simulink model "exampleModel_bus_axi"  (R2017b)
settings: Solver=VariableStepAuto  StartTime=0.0  StopTime=3e-5  RelTol=1e-3
PreLoadFcn:
  | setup
values from neighbouring files (symbols this model uses):
  axiClk = 156.25e6    (= 156250000)    [setup.m]    (also in setup_exampleModel_bus_axi_simulink.m; setup_exampleModel_bus_axi_simulink_lcls2.m; setup_lcls2_pcav.m; sysgen_signal.m)
  cav1p1_addr = 204    [setup_exampleModel_bus_axi_simulink.m]    (also in setup_exampleModel_bus_axi_simulink_lcls2.m; setup_lcls2_pcav.m; sysgen_signal.m)
  cav1p2_addr = cav1p1_addr * 2    (= 408)    [setup_exampleModel_bus_axi_simulink.m]    (also in setup_exampleModel_bus_axi_simulink_lcls2.m; setup_lcls2_pcav.m; sysgen_signal.m)
  cav2p1_addr = cav1p1_addr * 3    (= 612)    [setup_exampleModel_bus_axi_simulink.m]    (also in setup_exampleModel_bus_axi_simulink_lcls2.m; setup_lcls2_pcav.m; sysgen_signal.m)
  cav2p2_addr = cav1p1_addr * 4    (= 816)    [setup_exampleModel_bus_axi_simulink.m]    (also in setup_exampleModel_bus_axi_simulink_lcls2.m; setup_lcls2_pcav.m; sysgen_signal.m)
  Fadc = Fs/interleavedChannels    (= 29750000)    [setup.m]    (also in setup_exampleModel_bus_axi_simulink.m = 357000000; setup_exampleModel_bus_axi_simulink_lcls2.m = 351000000; setup_lcls2_pcav.m = 357000000; sysgen_signal.m = 357000000)
  Fproc = 204e6    (= 204000000)    [setup_exampleModel_bus_axi_simulink.m]    (also in setup_exampleModel_bus_axi_simulink_lcls2.m = 200571400; setup_lcls2_pcav.m; sysgen_signal.m)
  Fsig = Fproc/12    (= 17000000)    [setup_exampleModel_bus_axi_simulink.m]    (also in setup_exampleModel_bus_axi_simulink_lcls2.m = 16714283.3333; setup_lcls2_pcav.m)
  Tadc = 1/fadc    (= 2.80112044818e-09)    [cavity_signal.m]    (also in setup_exampleModel_bus_axi_simulink.m; setup_exampleModel_bus_axi_simulink_lcls2.m = 2.849002849e-09; setup_lcls2_pcav.m; setup_pcav_simulink.m)
undefined symbols (not defined in the file or in its folder): AXI4, Lite
libraries: xbsIndex_r4 x2037, llrf_lib x10, simulink x1
(part 6 of 12)

== system exampleModel_bus_axi/example/dsp/Cav1/Masking_n_delay ==
  note: delay for the comparison because Axilite register
      | takes a about 40 dsp clk cycles to load in
  phi_reset_trig : Inport
  start_pt : Inport  Port=2
  stop_pt : Inport  Port=3
  flo_start : Inport  Port=4
  flo_stop : Inport  Port=5
  Constant1 : xbsIndex_r4/Constant  const=0  gui_display_data_type=Fixed-point  arith_type=Unsigned  n_bits=16  bin_pt=0  preci_type=Single  exp_width=8  frac_width=24  explicit_period=off  period=1  equ=P=C  opselect=C  inp2=PCIN>>17  opr=+  inp1=P  carry=CIN  dbl_ovrd=off  block_type=constant
  Constant4 : xbsIndex_r4/Constant  const=0  gui_display_data_type=Fixed-point  arith_type=Unsigned  n_bits=1  bin_pt=0  preci_type=Single  exp_width=8  frac_width=24  explicit_period=off  period=1  equ=P=C  opselect=C  inp2=PCIN>>17  opr=+  inp1=P  carry=CIN  dbl_ovrd=off  block_type=constant
  Convert11 : xbsIndex_r4/Convert  gui_display_data_type=Fixed-point  arith_type=Unsigned  n_bits=1  bin_pt=0  float_type=Single  exp_bits=8  fraction_bits=24  quantization=Truncate  overflow=Wrap  en=off  latency=1  pipeline=off  dbl_ovrd=off  block_type=convert
  Convert2 : xbsIndex_r4/Convert  gui_display_data_type=Fixed-point  arith_type=Unsigned  n_bits=1  bin_pt=0  float_type=Single  exp_bits=8  fraction_bits=24  quantization=Truncate  overflow=Wrap  en=off  latency=1  pipeline=off  dbl_ovrd=off  block_type=convert
  Convert3 : xbsIndex_r4/Convert  gui_display_data_type=Boolean  arith_type=Boolean  n_bits=16  bin_pt=14  float_type=Single  exp_bits=8  fraction_bits=24  quantization=Truncate  overflow=Wrap  en=off  latency=1  pipeline=off  dbl_ovrd=off  block_type=convert
  Convert4 : xbsIndex_r4/Convert  gui_display_data_type=Fixed-point  arith_type=Unsigned  n_bits=8  bin_pt=0  float_type=Single  exp_bits=8  fraction_bits=24  quantization=Truncate  overflow=Saturate  en=off  latency=1  pipeline=off  dbl_ovrd=off  block_type=convert
  Convert7 : xbsIndex_r4/Convert  gui_display_data_type=Boolean  arith_type=Boolean  n_bits=1  bin_pt=0  float_type=Single  exp_bits=8  fraction_bits=24  quantization=Truncate  overflow=Wrap  en=off  latency=1  pipeline=off  dbl_ovrd=off  block_type=convert
  Convert8 : xbsIndex_r4/Convert  gui_display_data_type=Boolean  arith_type=Boolean  n_bits=1  bin_pt=0  float_type=Single  exp_bits=8  fraction_bits=24  quantization=Truncate  overflow=Wrap  en=off  latency=1  pipeline=off  dbl_ovrd=off  block_type=convert
  Counter : xbsIndex_r4/Counter  cnt_type=Count Limited  cnt_to=2^15  operation=Up  start_count=0  cnt_by_val=1  arith_type=Unsigned  n_bits=16  bin_pt=0  load_pin=off  rst=on  en=on  explicit_period=off  period=12/Fproc  use_behavioral_HDL=off  implementation=Fabric  dbl_ovrd=off  block_type=counter
  Delay{1..4} (4 alike) : xbsIndex_r4/Delay  rst=off  infoeditControl=Selection of Reset will increase slice count due to use of real FFs and instead of SRLs  en=off  latency=1  reg_retiming=off  dbl_ovrd=off  block_type=delay
  Delay6 : xbsIndex_r4/Delay  rst=off  infoeditControl=Selection of Reset will increase slice count due to use of real FFs and instead of SRLs  en=off  latency=2  reg_retiming=off  dbl_ovrd=off  block_type=delay
  Delay7 : xbsIndex_r4/Delay  rst=off  infoeditControl=Selection of Reset will increase slice count due to use of real FFs and instead of SRLs  en=off  latency=2  reg_retiming=off  dbl_ovrd=off  block_type=delay
  Down Sample{1..4} (4 alike) : xbsIndex_r4/Down Sample  sample_ratio=12  sample_phase="Last Value of Frame  (most efficient)"  en=off  rst=off  latency=1  dbl_ovrd=off  block_type=dsamp
  Logical1 : xbsIndex_r4/Logical  logical_function=AND  inputs=2  en=off  latency=1  precision=Full  arith_type=Unsigned  n_bits=16  bin_pt=0  align_bp=on  dbl_ovrd=off  block_type=logical
  Logical2 : xbsIndex_r4/Logical  logical_function=AND  inputs=2  en=off  latency=1  precision=Full  arith_type=Unsigned  n_bits=16  bin_pt=0  align_bp=on  dbl_ovrd=off  block_type=logical
  Register1 : xbsIndex_r4/Register  init=0  rst=off  en=on  dbl_ovrd=off  block_type=register
  Register10 : xbsIndex_r4/Register  init=0  rst=off  en=off  dbl_ovrd=off  block_type=register
  Register2 : xbsIndex_r4/Register  init=100  rst=off  en=off  dbl_ovrd=off  block_type=register
  Register3 : xbsIndex_r4/Register  init=100  rst=off  en=off  dbl_ovrd=off  block_type=register
  Register5 : xbsIndex_r4/Register  init=0  rst=off  en=off  dbl_ovrd=off  block_type=register
  Register6 : xbsIndex_r4/Register  init=100  rst=off  en=off  dbl_ovrd=off  block_type=register
  Relational1 : xbsIndex_r4/Relational  mode=a<b  op_type=Bool  en=on  latency=1  dbl_ovrd=off  block_type=relational
  Relational2 : xbsIndex_r4/Relational  mode=a>b  op_type=Bool  en=off  latency=1  dbl_ovrd=off  block_type=relational
  Relational3 : xbsIndex_r4/Relational  mode=a<b  op_type=Bool  en=on  latency=1  dbl_ovrd=off  block_type=relational
  Relational4 : xbsIndex_r4/Relational  mode=a>b  op_type=Bool  en=on  latency=1  dbl_ovrd=off  block_type=relational
  Relational6 : xbsIndex_r4/Relational  mode=a>b  op_type=Bool  en=on  latency=1  dbl_ovrd=off  block_type=relational
  Relational7 : xbsIndex_r4/Relational  mode=a>b  op_type=Bool  en=off  latency=1  dbl_ovrd=off  block_type=relational
  trig_reset : Outport
  counter : Outport  Port=2
  eval_window : Outport  Port=3
  flo_window : Outport  Port=4
  Stream_valid : Outport  Port=5
  wires:
  start_pt/1 -> Register5/1
  phi_reset_trig/1 -> Register10/1
  Register5/1 -> Down Sample1/1
  stop_pt/1 -> Register6/1
  Register6/1 -> Down Sample2/1
  Convert3/1 -> Register1/2, Register1/1, Counter/1, trig_reset/1
  Delay2/1 -> Relational4/2
  Delay3/1 -> Relational3/2
  Constant1/1 -> Relational2/2
  Relational3/1 -> Convert7/1
  Relational4/1 -> Convert8/1
  Logical1/1 -> Convert11/1
  Convert8/1 -> Logical1/1
  Convert7/1 -> Logical1/2
  Convert11/1 -> eval_window/1
  Relational2/1 -> [enb], Relational3/3, Relational4/3
  Counter/1 -> Convert4/1
  Down Sample1/1 -> Delay2/1
  Down Sample2/1 -> [stop], Delay3/1
  Delay1/1 -> Relational4/1
  Delay4/1 -> Relational3/1
  Delay7/1 -> Relational1/1
  flo_stop/1 -> Register3/1
  Logical2/1 -> Convert2/1
  Relational1/1 -> Logical2/2
  Convert2/1 -> flo_window/1
  Delay6/1 -> Relational6/1
  flo_start/1 -> Register2/1
  Relational6/1 -> Logical2/1
  Constant4/1 -> Relational7/2
  Relational7/1 -> Stream_valid/1
  Register10/1 -> Convert3/1
  Register1/1 -> Counter/2
  Convert4/1 -> [cntr], Relational7/1, counter/1
  [cntr] -> Relational2/1, Delay4/1, Delay1/1
  [cntr] -> Delay7/1, Delay6/1
  [enb] -> Relational6/3, Relational1/3
  Register2/1 -> Down Sample3/1
  Down Sample3/1 -> Relational6/2
  Down Sample4/1 -> Relational1/2
  Register3/1 -> Down Sample4/1

== system exampleModel_bus_axi/example/dsp/Cav1/PA_select ==
  PA_bus : Inport
  PA_chan_sel : Inport  Port=2
  Bus Creator3 : BusCreator  Inputs=3
  Bus Selector : BusSelector  OutputSignals=amp,phase,sync
  Bus Selector1 : BusSelector  OutputSignals=amp,phase,sync,channel
  Channel Select1 : llrf_lib/Sysgen/Single Rate/Channel Select  SystemSampleTime=-1
      settings: SourceProductName=LLRF Library
  Amp : Outport
  Phase : Outport  Port=2
  sync : Outport  Port=3
  wires:
  Bus Selector/3 -> sync/1  "<sync>"
  Bus Selector/2 -> Phase/1  "<phase>"
  Bus Selector/1 -> Amp/1  "<amp>"
  Bus Selector1/1 -> Channel Select1/1  "<amp>"
  Bus Selector1/2 -> Channel Select1/2  "<phase>"
  Bus Selector1/3 -> Channel Select1/3  "<sync>"
  Bus Selector1/4 -> Channel Select1/4  "<channel>"
  Channel Select1/1 -> Bus Creator3/1  "amp"
  Channel Select1/2 -> Bus Creator3/2  "phase"
  Channel Select1/3 -> Bus Creator3/3  "sync"
  Bus Creator3/1 -> Bus Selector/1
  PA_chan_sel/1 -> Channel Select1/5
  PA_bus/1 -> Bus Selector1/1

== system exampleModel_bus_axi/example/dsp/Cav1/PA_select1 ==
  PA_bus : Inport
  PA_chan_sel : Inport  Port=2
  Bus Creator3 : BusCreator  Inputs=3
  Bus Selector : BusSelector  OutputSignals=amp,phase,sync
  Bus Selector1 : BusSelector  OutputSignals=amp,phase,sync,channel
  Channel Select1 : llrf_lib/Sysgen/Single Rate/Channel Select  SystemSampleTime=-1
      settings: SourceProductName=LLRF Library
  Amp : Outport
  Phase : Outport  Port=2
  sync : Outport  Port=3
  wires:
  PA_bus/1 -> Bus Selector1/1
  PA_chan_sel/1 -> Channel Select1/5
  Bus Creator3/1 -> Bus Selector/1
  Channel Select1/3 -> Bus Creator3/3  "sync"
  Channel Select1/2 -> Bus Creator3/2  "phase"
  Channel Select1/1 -> Bus Creator3/1  "amp"
  Bus Selector1/4 -> Channel Select1/4  "<channel>"
  Bus Selector1/3 -> Channel Select1/3  "<sync>"
  Bus Selector1/2 -> Channel Select1/2  "<phase>"
  Bus Selector1/1 -> Channel Select1/1  "<amp>"
  Bus Selector/1 -> Amp/1  "<amp>"
  Bus Selector/2 -> Phase/1  "<phase>"
  Bus Selector/3 -> sync/1  "<sync>"

== system exampleModel_bus_axi/example/dsp/Cav1/Subsystem1 ==
  IQ_stream_in : Inport
  IQ_chan_sel : Inport  Port=2
  Bus Creator5 : BusCreator  Inputs=3
  Bus Selector : BusSelector  OutputSignals=ddcI,ddcQ,sync
  Bus Selector3 : BusSelector  OutputSignals=ddcI,ddcQ,ddcSync,ddcChannel
  Channel Select3 : llrf_lib/Sysgen/Single Rate/Channel Select  SystemSampleTime=-1
      settings: SourceProductName=LLRF Library
  ddcI : Outport
  ddcQ : Outport  Port=2
  sync : Outport  Port=3
  wires:
  IQ_stream_in/1 -> Bus Selector3/1
  IQ_chan_sel/1 -> Channel Select3/5
  Channel Select3/3 -> Bus Creator5/3  "sync"
  Bus Selector3/2 -> Channel Select3/2  "<ddcQ>"
  Channel Select3/1 -> Bus Creator5/1  "ddcI"
  Channel Select3/2 -> Bus Creator5/2  "ddcQ"
  Bus Selector3/1 -> Channel Select3/1  "<ddcI>"
  Bus Selector3/4 -> Channel Select3/4  "<ddcChannel>"
  Bus Selector3/3 -> Channel Select3/3  "<ddcSync>"
  Bus Creator5/1 -> Bus Selector/1
  Bus Selector/1 -> ddcI/1  "<ddcI>"
  Bus Selector/2 -> ddcQ/1  "<ddcQ>"
  Bus Selector/3 -> sync/1  "<sync>"

== system exampleModel_bus_axi/example/dsp/Cav1/Subsystem10 ==
  d : Inport
  reset : Inport  Port=2
  cntr : Inport  Port=3
  threshold : Inport  Port=4
  Register11 : xbsIndex_r4/Register  init=0  rst=on  en=on  dbl_ovrd=off  block_type=register
  Relational4 : xbsIndex_r4/Relational  mode=a>b  op_type=Bool  en=off  latency=1  dbl_ovrd=off  block_type=relational
  posedge_pulse : Subsystem
  q : Outport
  wires:
  threshold/1 -> Relational4/2
  reset/1 -> Register11/2
  Relational4/1 -> posedge_pulse/1(In1)
  posedge_pulse/1(Out1) -> Register11/3
  Register11/1 -> q/1
  cntr/1 -> Relational4/1
  d/1 -> Register11/1

== system exampleModel_bus_axi/example/dsp/Cav1/Subsystem11 ==
  d : Inport
  reset : Inport  Port=2
  cntr : Inport  Port=3
  threshold : Inport  Port=4
  Register11 : xbsIndex_r4/Register  init=0  rst=on  en=on  dbl_ovrd=off  block_type=register
  Relational4 : xbsIndex_r4/Relational  mode=a>b  op_type=Bool  en=off  latency=1  dbl_ovrd=off  block_type=relational
  posedge_pulse : Subsystem
  q : Outport
  wires:
  d/1 -> Register11/1
  cntr/1 -> Relational4/1
  Register11/1 -> q/1
  posedge_pulse/1(Out1) -> Register11/3
  Relational4/1 -> posedge_pulse/1(In1)
  reset/1 -> Register11/2
  threshold/1 -> Relational4/2

== system exampleModel_bus_axi/example/dsp/Cav1/Subsystem12 ==
  d : Inport
  reset : Inport  Port=2
  cntr : Inport  Port=3
  threshold : Inport  Port=4
  Register11 : xbsIndex_r4/Register  init=0  rst=on  en=on  dbl_ovrd=off  block_type=register
  Relational4 : xbsIndex_r4/Relational  mode=a>b  op_type=Bool  en=off  latency=1  dbl_ovrd=off  block_type=relational
  posedge_pulse : Subsystem
  q : Outport
  wires:
  threshold/1 -> Relational4/2
  reset/1 -> Register11/2
  Relational4/1 -> posedge_pulse/1(In1)
  posedge_pulse/1(Out1) -> Register11/3
  Register11/1 -> q/1
  cntr/1 -> Relational4/1
  d/1 -> Register11/1

== system exampleModel_bus_axi/example/dsp/Cav1/Subsystem13 ==
  d : Inport
  reset : Inport  Port=2
  cntr : Inport  Port=3
  threshold : Inport  Port=4
  Register11 : xbsIndex_r4/Register  init=0  rst=on  en=on  dbl_ovrd=off  block_type=register
  Relational4 : xbsIndex_r4/Relational  mode=a>b  op_type=Bool  en=off  latency=1  dbl_ovrd=off  block_type=relational
  posedge_pulse : Subsystem
  q : Outport
  wires:
  d/1 -> Register11/1
  cntr/1 -> Relational4/1
  Register11/1 -> q/1
  posedge_pulse/1(Out1) -> Register11/3
  Relational4/1 -> posedge_pulse/1(In1)
  reset/1 -> Register11/2
  threshold/1 -> Relational4/2

== system exampleModel_bus_axi/example/dsp/Cav1/Subsystem14 ==
  d : Inport
  reset : Inport  Port=2
  cntr : Inport  Port=3
  threshold : Inport  Port=4
  Register11 : xbsIndex_r4/Register  init=0  rst=on  en=on  dbl_ovrd=off  block_type=register
  Relational4 : xbsIndex_r4/Relational  mode=a>b  op_type=Bool  en=off  latency=1  dbl_ovrd=off  block_type=relational
  posedge_pulse : Subsystem
  q : Outport
  wires:
  threshold/1 -> Relational4/2
  reset/1 -> Register11/2
  Relational4/1 -> posedge_pulse/1(In1)
  posedge_pulse/1(Out1) -> Register11/3
  Register11/1 -> q/1
  cntr/1 -> Relational4/1
  d/1 -> Register11/1

== system exampleModel_bus_axi/example/dsp/Cav1/Subsystem2 ==
  d : Inport
  reset : Inport  Port=2
  cntr : Inport  Port=3
  threshold : Inport  Port=4
  Register11 : xbsIndex_r4/Register  init=0  rst=on  en=on  dbl_ovrd=off  block_type=register
  Relational4 : xbsIndex_r4/Relational  mode=a>b  op_type=Bool  en=off  latency=1  dbl_ovrd=off  block_type=relational
  posedge_pulse : Subsystem
  q : Outport
  wires:
  d/1 -> Register11/1
  cntr/1 -> Relational4/1
  Register11/1 -> q/1
  posedge_pulse/1(Out1) -> Register11/3
  Relational4/1 -> posedge_pulse/1(In1)
  reset/1 -> Register11/2
  threshold/1 -> Relational4/2

== system exampleModel_bus_axi/example/dsp/Cav1/Subsystem3 ==
  IQ_stream_in : Inport
  IQ_chan_sel : Inport  Port=2
  Bus Creator5 : BusCreator  Inputs=3
  Bus Selector : BusSelector  OutputSignals=ddcI,ddcQ,sync
  Bus Selector3 : BusSelector  OutputSignals=ddcI,ddcQ,ddcSync,ddcChannel
  Channel Select3 : llrf_lib/Sysgen/Single Rate/Channel Select  SystemSampleTime=-1
      settings: SourceProductName=LLRF Library
  ddcI : Outport
  ddcQ : Outport  Port=2
  sync : Outport  Port=3
  wires:
  Bus Selector/3 -> sync/1  "<sync>"
  Bus Selector/2 -> ddcQ/1  "<ddcQ>"
  Bus Selector/1 -> ddcI/1  "<ddcI>"
  Bus Creator5/1 -> Bus Selector/1
  Bus Selector3/3 -> Channel Select3/3  "<ddcSync>"
  Bus Selector3/4 -> Channel Select3/4  "<ddcChannel>"
  Bus Selector3/1 -> Channel Select3/1  "<ddcI>"
  Channel Select3/2 -> Bus Creator5/2  "ddcQ"
  Channel Select3/1 -> Bus Creator5/1  "ddcI"
  Bus Selector3/2 -> Channel Select3/2  "<ddcQ>"
  Channel Select3/3 -> Bus Creator5/3  "sync"
  IQ_chan_sel/1 -> Channel Select3/5
  IQ_stream_in/1 -> Bus Selector3/1

== system exampleModel_bus_axi/example/dsp/Cav1/Subsystem4 ==
  d : Inport
  reset : Inport  Port=2
  cntr : Inport  Port=3
  threshold : Inport  Port=4
  Gateway Out{1,7..9} (4 alike) : xbsIndex_r4/Gateway Out  inherit_from_input=off  hdl_port=on  rows=1  columns=1  UseAsDAC=off  DACChannel='1'  interface=None  automatic_assignment=on  address_offset=hex2dec('00')  intf_name=''  intf_description=''  timing_constraint=None  locs_specified=off  LOCs={}  io_standard={}  block_type=gatewayout
  Register11 : xbsIndex_r4/Register  init=0  rst=on  en=on  dbl_ovrd=off  block_type=register
  Relational4 : xbsIndex_r4/Relational  mode=a>b  op_type=Bool  en=off  latency=1  dbl_ovrd=off  block_type=relational
  Scope3 : Scope  NumInputPorts=4
  posedge_pulse : Subsystem
  q : Outport
  wires:
  d/1 -> Gateway Out7/1, Register11/1
  cntr/1 -> Relational4/1
  Register11/1 -> Gateway Out8/1, q/1
  posedge_pulse/1(Out1) -> Register11/3, Gateway Out1/1
  Relational4/1 -> posedge_pulse/1(In1)
  reset/1 -> Gateway Out9/1, Register11/2
  threshold/1 -> Relational4/2
  Gateway Out1/1 -> Scope3/4
  Gateway Out7/1 -> Scope3/1
  Gateway Out8/1 -> Scope3/2
  Gateway Out9/1 -> Scope3/3

== system exampleModel_bus_axi/example/dsp/Cav1/Subsystem5 ==
  d : Inport
  reset : Inport  Port=2
  cntr : Inport  Port=3
  threshold : Inport  Port=4
  Register11 : xbsIndex_r4/Register  init=0  rst=on  en=on  dbl_ovrd=off  block_type=register
  Relational4 : xbsIndex_r4/Relational  mode=a>b  op_type=Bool  en=off  latency=1  dbl_ovrd=off  block_type=relational
  posedge_pulse : Subsystem
  q : Outport
  wires:
  threshold/1 -> Relational4/2
  reset/1 -> Register11/2
  Relational4/1 -> posedge_pulse/1(In1)
  posedge_pulse/1(Out1) -> Register11/3
  Register11/1 -> q/1
  cntr/1 -> Relational4/1
  d/1 -> Register11/1

== system exampleModel_bus_axi/example/dsp/Cav1/Subsystem6 ==
  d : Inport
  reset : Inport  Port=2
  cntr : Inport  Port=3
  threshold : Inport  Port=4
  Register11 : xbsIndex_r4/Register  init=0  rst=on  en=on  dbl_ovrd=off  block_type=register
  Relational4 : xbsIndex_r4/Relational  mode=a>b  op_type=Bool  en=off  latency=1  dbl_ovrd=off  block_type=relational
  posedge_pulse : Subsystem
  q : Outport
  wires:
  threshold/1 -> Relational4/2
  reset/1 -> Register11/2
  Relational4/1 -> posedge_pulse/1(In1)
  posedge_pulse/1(Out1) -> Register11/3
  Register11/1 -> q/1
  cntr/1 -> Relational4/1
  d/1 -> Register11/1

== system exampleModel_bus_axi/example/dsp/Cav1/Subsystem7 ==
  d : Inport
  reset : Inport  Port=2
  cntr : Inport  Port=3
  threshold : Inport  Port=4
  Register11 : xbsIndex_r4/Register  init=0  rst=on  en=on  dbl_ovrd=off  block_type=register
  Relational4 : xbsIndex_r4/Relational  mode=a>b  op_type=Bool  en=off  latency=1  dbl_ovrd=off  block_type=relational
  posedge_pulse : Subsystem
  q : Outport
  wires:
  d/1 -> Register11/1
  cntr/1 -> Relational4/1
  Register11/1 -> q/1
  posedge_pulse/1(Out1) -> Register11/3
  Relational4/1 -> posedge_pulse/1(In1)
  reset/1 -> Register11/2
  threshold/1 -> Relational4/2

== system exampleModel_bus_axi/example/dsp/Cav1/Subsystem8 ==
  d : Inport
  reset : Inport  Port=2
  cntr : Inport  Port=3
  threshold : Inport  Port=4
  Register11 : xbsIndex_r4/Register  init=0  rst=on  en=on  dbl_ovrd=off  block_type=register
  Relational4 : xbsIndex_r4/Relational  mode=a>b  op_type=Bool  en=off  latency=1  dbl_ovrd=off  block_type=relational
  posedge_pulse : Subsystem
  q : Outport
  wires:
  threshold/1 -> Relational4/2
  reset/1 -> Register11/2
  Relational4/1 -> posedge_pulse/1(In1)
  posedge_pulse/1(Out1) -> Register11/3
  Register11/1 -> q/1
  cntr/1 -> Relational4/1
  d/1 -> Register11/1

== system exampleModel_bus_axi/example/dsp/Cav1/Subsystem9 ==
  d : Inport
  reset : Inport  Port=2
  cntr : Inport  Port=3
  threshold : Inport  Port=4
  Register11 : xbsIndex_r4/Register  init=0  rst=on  en=on  dbl_ovrd=off  block_type=register
  Relational4 : xbsIndex_r4/Relational  mode=a>b  op_type=Bool  en=off  latency=1  dbl_ovrd=off  block_type=relational
  posedge_pulse : Subsystem
  q : Outport
  wires:
  d/1 -> Register11/1
  cntr/1 -> Relational4/1
  Register11/1 -> q/1
  posedge_pulse/1(Out1) -> Register11/3
  Relational4/1 -> posedge_pulse/1(In1)
  reset/1 -> Register11/2
  threshold/1 -> Relational4/2

== system exampleModel_bus_axi/example/dsp/Cav1/c1p1_Masking_window ==
  note: delay for the comparison because Axilite register
      | takes a about 40 dsp clk cycles to load in
  counter : Inport
  start_pt : Inport  Port=2
  stop_pt : Inport  Port=3
  Constant1 : xbsIndex_r4/Constant  const=0  gui_display_data_type=Fixed-point  arith_type=Unsigned  n_bits=16  bin_pt=0  preci_type=Single  exp_width=8  frac_width=24  explicit_period=off  period=1  equ=P=C  opselect=C  inp2=PCIN>>17  opr=+  inp1=P  carry=CIN  dbl_ovrd=off  block_type=constant
  Convert11 : xbsIndex_r4/Convert  gui_display_data_type=Fixed-point  arith_type=Unsigned  n_bits=1  bin_pt=0  float_type=Single  exp_bits=8  fraction_bits=24  quantization=Truncate  overflow=Wrap  en=off  latency=1  pipeline=off  dbl_ovrd=off  block_type=convert
  Delay{1..4} (4 alike) : xbsIndex_r4/Delay  rst=off  infoeditControl=Selection of Reset will increase slice count due to use of real FFs and instead of SRLs  en=off  latency=1  reg_retiming=off  dbl_ovrd=off  block_type=delay
  Down Sample1 : xbsIndex_r4/Down Sample  sample_ratio=12  sample_phase="Last Value of Frame  (most efficient)"  en=off  rst=off  latency=1  dbl_ovrd=off  block_type=dsamp
  Down Sample2 : xbsIndex_r4/Down Sample  sample_ratio=12  sample_phase="Last Value of Frame  (most efficient)"  en=off  rst=off  latency=1  dbl_ovrd=off  block_type=dsamp
  Logical1 : xbsIndex_r4/Logical  logical_function=AND  inputs=2  en=off  latency=1  precision=Full  arith_type=Unsigned  n_bits=16  bin_pt=0  align_bp=on  dbl_ovrd=off  block_type=logical
  Register5 : xbsIndex_r4/Register  init=0  rst=off  en=off  dbl_ovrd=off  block_type=register
  Register6 : xbsIndex_r4/Register  init=100  rst=off  en=off  dbl_ovrd=off  block_type=register
  Relational2 : xbsIndex_r4/Relational  mode=a>b  op_type=Bool  en=off  latency=1  dbl_ovrd=off  block_type=relational
  Relational3 : xbsIndex_r4/Relational  mode=a<b  op_type=Bool  en=on  latency=1  dbl_ovrd=off  block_type=relational
  Relational4 : xbsIndex_r4/Relational  mode=a>b  op_type=Bool  en=on  latency=1  dbl_ovrd=off  block_type=relational
  eval_window : Outport
  wires:
  start_pt/1 -> Register5/1
  Register5/1 -> Down Sample1/1
  stop_pt/1 -> Register6/1
  Register6/1 -> Down Sample2/1
  Delay2/1 -> Relational4/2
  Delay3/1 -> [stop], Relational3/2
  Constant1/1 -> Relational2/2
  Logical1/1 -> Convert11/1
  Relational3/1 -> Logical1/2
  Convert11/1 -> eval_window/1
  Relational2/1 -> [enb], Relational3/3, Relational4/3
  counter/1 -> [cntr]
  Down Sample1/1 -> Delay2/1
  Down Sample2/1 -> Delay3/1
  Delay1/1 -> Relational4/1
  Delay4/1 -> Relational3/1
  Relational4/1 -> Logical1/1
  [cntr] -> Relational2/1, Delay1/1, Delay4/1

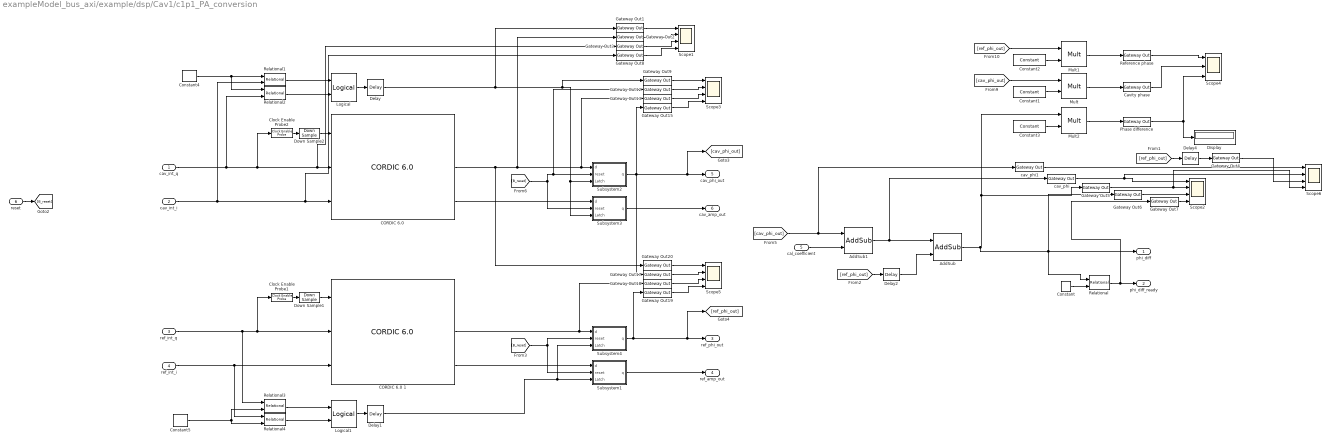
== system exampleModel_bus_axi/example/dsp/Cav1/c1p1_PA_conversion ==
  cav_int_q : Inport
  cav_int_i : Inport  Port=2
  ref_int_q : Inport  Port=3
  ref_int_i : Inport  Port=4
  cal_coefficient : Inport  Port=5
  reset : Inport  Port=6
  AddSub : xbsIndex_r4/AddSub  mode=Subtraction  use_carryin=off  use_carryout=off  en=off  latency=1  precision=User Defined  arith_type="Signed  (2's comp)"  n_bits=18  bin_pt=15  quantization=Truncate  overflow=Wrap  use_behavioral_HDL=off  hw_selection=Fabric  pipelined=off  dbl_ovrd=off  block_type=addsub
  AddSub1 : xbsIndex_r4/AddSub  mode=Addition  use_carryin=off  use_carryout=off  en=off  latency=1  precision=User Defined  arith_type="Signed  (2's comp)"  n_bits=18  bin_pt=15  quantization=Truncate  overflow=Wrap  use_behavioral_HDL=off  hw_selection=Fabric  pipelined=off  dbl_ovrd=off  block_type=addsub
  "CORDIC 6.0 " : xbsIndex_r4/CORDIC 6.0   functional_selection=Translate  architectural_configuration=Parallel  pipelining_mode=Maximum  data_format=SignedFraction  phase_format=Scaled_Radians  input_width=18  output_width=18  round_mode=Truncate  iterations=0  precision=0  compensation_scaling=No_Scale_Compensation  coarse_rotation=on  aclken=off  aresetn=off  out_tready=off  cartesian_has_tuser=off  cartesian_has_tlast=off  cartesian_tuser_width=1  phase_has_tuser=off  phase_has_tlast=off  phase_tuser_width=1  out_tlast_behv=Null  flow_control=NonBlocking  optimize_goal=Resources  trim_axipin_name=on  simulation_type=hybrid_sim  simulation_model=sysgen:cordic_v6_0  data_path_portlist={'s_axis_cartesian_tdata_imag', 's_axis_cartesian_tdata_real', 's_axis_phase_tdata_phase', 'm_axis_dout_tdata_imag', 'm_axis_dout_tdata_real', 'm_axis_dout_tdata_phase','m_axis_dout_tdata'}  ip_name=CORDIC  ip_version=6.0  dsptool_ready=true  ipcore_usecache=true  ipcore_useipmodelcache=true  wrapper_available=true  port_translation_map={ 'aclken' => 'en', 'aresetn' => 'rst' }  block_type=cordic_v6_0
      settings: infoedit=CORDIC 6.0
  CORDIC 6.0 1 : xbsIndex_r4/CORDIC 6.0   functional_selection=Translate  architectural_configuration=Parallel  pipelining_mode=Maximum  data_format=SignedFraction  phase_format=Scaled_Radians  input_width=18  output_width=18  round_mode=Truncate  iterations=0  precision=0  compensation_scaling=No_Scale_Compensation  coarse_rotation=on  aclken=off  aresetn=off  out_tready=off  cartesian_has_tuser=off  cartesian_has_tlast=off  cartesian_tuser_width=1  phase_has_tuser=off  phase_has_tlast=off  phase_tuser_width=1  out_tlast_behv=Null  flow_control=NonBlocking  optimize_goal=Resources  trim_axipin_name=on  simulation_type=hybrid_sim  simulation_model=sysgen:cordic_v6_0  data_path_portlist={'s_axis_cartesian_tdata_imag', 's_axis_cartesian_tdata_real', 's_axis_phase_tdata_phase', 'm_axis_dout_tdata_imag', 'm_axis_dout_tdata_real', 'm_axis_dout_tdata_phase','m_axis_dout_tdata'}  ip_name=CORDIC  ip_version=6.0  dsptool_ready=true  ipcore_usecache=true  ipcore_useipmodelcache=true  wrapper_available=true  port_translation_map={ 'aclken' => 'en', 'aresetn' => 'rst' }  block_type=cordic_v6_0
      settings: infoedit=CORDIC 6.0
  Cavity phase : xbsIndex_r4/Gateway Out  inherit_from_input=off  hdl_port=off  rows=1  columns=1  UseAsDAC=off  DACChannel='1'  interface=None  automatic_assignment=on  address_offset=hex2dec('00')  intf_name=''  intf_description=''  timing_constraint=None  locs_specified=off  LOCs={}  io_standard={}  block_type=gatewayout
  Clock Enable Probe1 : xbsIndex_r4/Clock Enable Probe  inherit_constraints=on  block_type=ceprobe
      settings: infoedit="Clock enable extractor.  Produces a Boolean output that mirrors the hardware clock enable associated with the input sample rate.<br><br>Hardware notes: in hardware this block costs nothing."
  Clock Enable Probe2 : xbsIndex_r4/Clock Enable Probe  inherit_constraints=on  block_type=ceprobe
      settings: infoedit="Clock enable extractor.  Produces a Boolean output that mirrors the hardware clock enable associated with the input sample rate.<br><br>Hardware notes: in hardware this block costs nothing."
  Constant : xbsIndex_r4/Constant  const=0  gui_display_data_type=Fixed-point  arith_type=Signed (2's comp)  n_bits=1  bin_pt=0  preci_type=Single  exp_width=8  frac_width=24  explicit_period=off  period=1  equ=P=C  opselect=C  inp2=PCIN>>17  opr=+  inp1=P  carry=CIN  dbl_ovrd=off  block_type=constant
  Constant1 : xbsIndex_r4/Constant  const=pi  gui_display_data_type=Fixed-point  arith_type=Unsigned  n_bits=16  bin_pt=14  preci_type=Single  exp_width=8  frac_width=24  explicit_period=off  period=1  equ=P=C  opselect=C  inp2=PCIN>>17  opr=+  inp1=P  carry=CIN  dbl_ovrd=off  block_type=constant
  Constant2 : xbsIndex_r4/Constant  const=pi  gui_display_data_type=Fixed-point  arith_type=Unsigned  n_bits=16  bin_pt=14  preci_type=Single  exp_width=8  frac_width=24  explicit_period=off  period=1  equ=P=C  opselect=C  inp2=PCIN>>17  opr=+  inp1=P  carry=CIN  dbl_ovrd=off  block_type=constant
  Constant3 : xbsIndex_r4/Constant  const=pi  gui_display_data_type=Fixed-point  arith_type=Unsigned  n_bits=16  bin_pt=14  preci_type=Single  exp_width=8  frac_width=24  explicit_period=off  period=1  equ=P=C  opselect=C  inp2=PCIN>>17  opr=+  inp1=P  carry=CIN  dbl_ovrd=off  block_type=constant
  Constant4 : xbsIndex_r4/Constant  const=0  gui_display_data_type=Fixed-point  arith_type=Signed (2's comp)  n_bits=16  bin_pt=14  preci_type=Single  exp_width=8  frac_width=24  explicit_period=off  period=1  equ=P=C  opselect=C  inp2=PCIN>>17  opr=+  inp1=P  carry=CIN  dbl_ovrd=off  block_type=constant
  Constant5 : xbsIndex_r4/Constant  const=0  gui_display_data_type=Fixed-point  arith_type=Signed (2's comp)  n_bits=16  bin_pt=14  preci_type=Single  exp_width=8  frac_width=24  explicit_period=off  period=1  equ=P=C  opselect=C  inp2=PCIN>>17  opr=+  inp1=P  carry=CIN  dbl_ovrd=off  block_type=constant
  Delay : xbsIndex_r4/Delay  rst=off  infoeditControl=Selection of Reset will increase slice count due to use of real FFs and instead of SRLs  en=off  latency=21  reg_retiming=off  dbl_ovrd=off  block_type=delay
  Delay1 : xbsIndex_r4/Delay  rst=off  infoeditControl=Selection of Reset will increase slice count due to use of real FFs and instead of SRLs  en=off  latency=21  reg_retiming=off  dbl_ovrd=off  block_type=delay
  Delay2 : xbsIndex_r4/Delay  rst=off  infoeditControl=Selection of Reset will increase slice count due to use of real FFs and instead of SRLs  en=off  latency=1  reg_retiming=off  dbl_ovrd=off  block_type=delay
  Delay4 : xbsIndex_r4/Delay  rst=off  infoeditControl=Selection of Reset will increase slice count due to use of real FFs and instead of SRLs  en=off  latency=1  reg_retiming=off  dbl_ovrd=off  block_type=delay
  Display : Display
  Down Sample1 : xbsIndex_r4/Down Sample  sample_ratio=12  sample_phase="Last Value of Frame  (most efficient)"  en=off  rst=off  latency=1  dbl_ovrd=off  block_type=dsamp
  Down Sample2 : xbsIndex_r4/Down Sample  sample_ratio=12  sample_phase="Last Value of Frame  (most efficient)"  en=off  rst=off  latency=1  dbl_ovrd=off  block_type=dsamp
  Gateway Out{1..9,12..13,15,17..20} (16 alike) : xbsIndex_r4/Gateway Out  inherit_from_input=off  hdl_port=off  rows=1  columns=1  UseAsDAC=off  DACChannel='1'  interface=None  automatic_assignment=on  address_offset=hex2dec('00')  intf_name=''  intf_description=''  timing_constraint=None  locs_specified=off  LOCs={}  io_standard={}  block_type=gatewayout
  Logical : xbsIndex_r4/Logical  logical_function=AND  inputs=2  en=off  latency=1  precision=Full  arith_type=Unsigned  n_bits=16  bin_pt=0  align_bp=on  dbl_ovrd=off  block_type=logical
  Logical1 : xbsIndex_r4/Logical  logical_function=AND  inputs=2  en=off  latency=1  precision=Full  arith_type=Unsigned  n_bits=16  bin_pt=0  align_bp=on  dbl_ovrd=off  block_type=logical
  Mult : xbsIndex_r4/Mult  precision=Full  arith_type="Signed  (2's comp)"  n_bits=16  bin_pt=14  quantization=Truncate  overflow=Wrap  en=off  latency=3  use_behavioral_HDL=off  opt=Speed  use_embedded=on  optimum_pipeline=off  pipeline=on  dbl_ovrd=off  use_rpm=on  placement_style=Triangular  block_type=mult
  Mult1 : xbsIndex_r4/Mult  precision=Full  arith_type="Signed  (2's comp)"  n_bits=16  bin_pt=14  quantization=Truncate  overflow=Wrap  en=off  latency=3  use_behavioral_HDL=off  opt=Speed  use_embedded=on  optimum_pipeline=off  pipeline=on  dbl_ovrd=off  use_rpm=on  placement_style=Triangular  block_type=mult
  Mult2 : xbsIndex_r4/Mult  precision=Full  arith_type="Signed  (2's comp)"  n_bits=16  bin_pt=14  quantization=Truncate  overflow=Wrap  en=off  latency=3  use_behavioral_HDL=off  opt=Speed  use_embedded=on  optimum_pipeline=off  pipeline=on  dbl_ovrd=off  use_rpm=on  placement_style=Triangular  block_type=mult
  Phase difference : xbsIndex_r4/Gateway Out  inherit_from_input=off  hdl_port=off  rows=1  columns=1  UseAsDAC=off  DACChannel='1'  interface=None  automatic_assignment=on  address_offset=hex2dec('00')  intf_name=''  intf_description=''  timing_constraint=None  locs_specified=off  LOCs={}  io_standard={}  block_type=gatewayout
  Reference phase : xbsIndex_r4/Gateway Out  inherit_from_input=off  hdl_port=off  rows=1  columns=1  UseAsDAC=off  DACChannel='1'  interface=None  automatic_assignment=on  address_offset=hex2dec('00')  intf_name=''  intf_description=''  timing_constraint=None  locs_specified=off  LOCs={}  io_standard={}  block_type=gatewayout
  Relational{,1..4} (5 alike) : xbsIndex_r4/Relational  mode=a!=b  op_type=Bool  en=off  latency=1  dbl_ovrd=off  block_type=relational
  Scope{1..3,5..6} (5 alike) : Scope  NumInputPorts=4
  Scope4 : Scope  NumInputPorts=3
  Subsystem1 : Subsystem
  Subsystem2 : Subsystem
  Subsystem3 : Subsystem
  Subsystem4 : Subsystem
  cav_phi : xbsIndex_r4/Gateway Out  inherit_from_input=off  hdl_port=off  rows=1  columns=1  UseAsDAC=off  DACChannel='1'  interface=None  automatic_assignment=on  address_offset=hex2dec('00')  intf_name=''  intf_description=''  timing_constraint=None  locs_specified=off  LOCs={}  io_standard={}  block_type=gatewayout
  cav_phi1 : xbsIndex_r4/Gateway Out  inherit_from_input=off  hdl_port=off  rows=1  columns=1  UseAsDAC=off  DACChannel='1'  interface=None  automatic_assignment=on  address_offset=hex2dec('00')  intf_name=''  intf_description=''  timing_constraint=None  locs_specified=off  LOCs={}  io_standard={}  block_type=gatewayout
  phi_diff : Outport
  phi_diff_ready : Outport  Port=2
  ref_phi_out : Outport  Port=3
  ref_amp_out : Outport  Port=4
  cav_phi_out : Outport  Port=5
  cav_amp_out : Outport  Port=6
  wires:
  ref_int_i/1 -> CORDIC 6.0 1/3, Relational4/1
  ref_int_q/1 -> Relational3/1, CORDIC 6.0 1/2, Clock Enable Probe1/1
  [ref_phi_out] -> Delay4/1
  AddSub1/1 -> cav_phi/1, AddSub/1
  [cav_phi_out] -> cav_phi1/1, AddSub1/1
  cal_coefficient/1 -> AddSub1/2
  Subsystem4/1(q) -> Gateway Out19/1, [ref_phi_out], ref_phi_out/1
  Subsystem1/1(q) -> ref_amp_out/1
  Subsystem2/1(q) -> Gateway Out17/1, Gateway Out15/1, [cav_phi_out], cav_phi_out/1
  Subsystem3/1(q) -> cav_amp_out/1
  reset/1 -> [B_reset]
  [B_reset] -> Subsystem4/2(reset), Subsystem1/2(reset)
  [B_reset] -> Subsystem3/2(reset), Gateway Out12/1, Subsystem2/2(reset)
  AddSub/1 -> Gateway Out6/1, phi_diff/1, Relational/1, Mult2/1, Gateway Out5/1
  Delay2/1 -> AddSub/2
  Gateway Out5/1 -> Scope6/4, Scope2/2
  cav_phi/1 -> Scope6/2, Scope2/1
  Gateway Out6/1 -> Scope2/3
  Gateway Out7/1 -> Scope2/4
  Constant/1 -> Relational/2
  Relational/1 -> Gateway Out7/1, phi_diff_ready/1
  Constant1/1 -> Mult/2
  [cav_phi_out] -> Mult/1
  [ref_phi_out] -> Mult1/1
  Constant2/1 -> Mult1/2
  Mult1/1 -> Reference phase/1
  Mult/1 -> Cavity phase/1
  Mult2/1 -> Phase difference/1
  Constant3/1 -> Mult2/2
  Cavity phase/1 -> Scope4/2
  Reference phase/1 -> Scope4/1
  Phase difference/1 -> Display/1, Scope4/3
  Clock Enable Probe2/1 -> Down Sample2/1
  Down Sample2/1 -> "CORDIC 6.0 "/1
  cav_int_q/1 -> Relational2/2, Clock Enable Probe2/1, Gateway Out3/1, "CORDIC 6.0 "/2
  Logical/1 -> Delay/1
  Relational2/1 -> Logical/2
  Relational1/1 -> Logical/1
  cav_int_i/1 -> Relational1/2, Gateway Out8/1, "CORDIC 6.0 "/3
  Constant4/1 -> Relational2/1, Relational1/1
  Delay/1 -> Gateway Out1/1, Gateway Out9/1, Subsystem3/3(Latch), Subsystem2/3(Latch)
  Clock Enable Probe1/1 -> Down Sample1/1
  Down Sample1/1 -> CORDIC 6.0 1/1
  Delay1/1 -> Subsystem4/3(Latch), Subsystem1/3(Latch)
  Relational3/1 -> Logical1/1
  Relational4/1 -> Logical1/2
  Logical1/1 -> Delay1/1
  Constant5/1 -> Relational4/2, Relational3/2
  CORDIC 6.0 1/3 -> Subsystem1/1(d)
  CORDIC 6.0 1/2 -> Gateway Out18/1, Subsystem4/1(d)
  "CORDIC 6.0 "/2 -> Gateway Out20/1, Gateway Out2/1, Gateway Out13/1, Subsystem2/1(d)
  "CORDIC 6.0 "/3 -> Subsystem3/1(d)
  Gateway Out8/1 -> Scope1/4
  Gateway Out3/1 -> Scope1/3
  Gateway Out1/1 -> Scope1/1
  Gateway Out2/1 -> Scope1/2
  Gateway Out12/1 -> Scope3/2
  Gateway Out9/1 -> Scope3/1
  Gateway Out13/1 -> Scope3/3
  Gateway Out15/1 -> Scope3/4
  Gateway Out19/1 -> Scope5/4
  Gateway Out18/1 -> Scope5/3
  Gateway Out20/1 -> Scope5/1
  Gateway Out17/1 -> Scope5/2
  cav_phi1/1 -> Scope6/1
  Delay4/1 -> Gateway Out4/1
  Gateway Out4/1 -> Scope6/3
  [ref_phi_out] -> Delay2/1
